simulink model "FTD_test_tau_w"  (R2023a)
settings: Solver=VariableStepAuto  StartTime=0.0  StopTime=150  FixedStep=0.002s  RelTol=1e-3
libraries: simulink x2
settings Model: Creator=邓宇飞  LastModifiedBy=邓宇飞

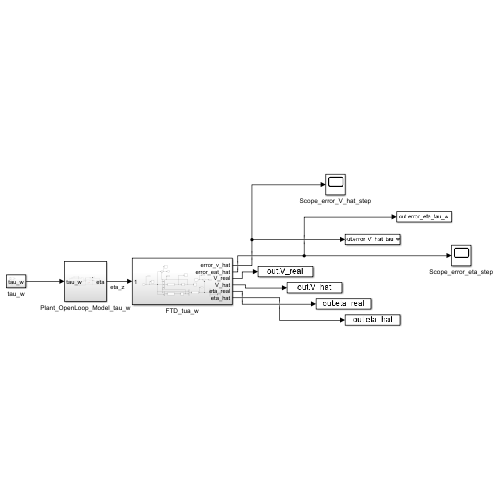
[thumbnail: Simulink's stored preview of the top-level diagram]
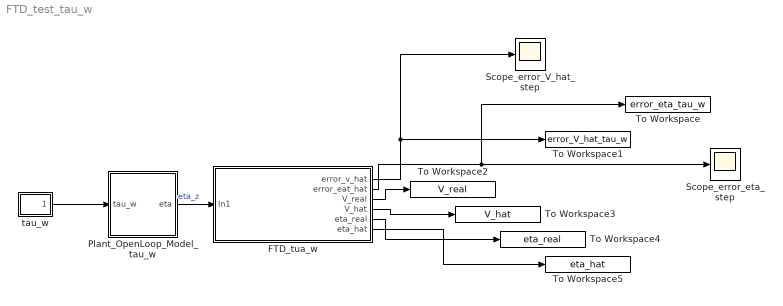
== system FTD_test_tau_w ==
  FTD_tua_w : Subsystem
  Plant_OpenLoop_Model_tau_w : Subsystem
  Scope_error_V_hat_step : Scope
  Scope_error_eta_step : Scope
  To Workspace : ToWorkspace  VariableName=error_eta_tau_w  SaveFormat=Timeseries  SampleTime=-1
  To Workspace1 : ToWorkspace  VariableName=error_V_hat_tau_w  SaveFormat=Timeseries  SampleTime=-1
  To Workspace2 : ToWorkspace  VariableName=V_real  SaveFormat=Timeseries  SampleTime=-1
  To Workspace3 : ToWorkspace  VariableName=V_hat  SaveFormat=Timeseries  SampleTime=-1
  To Workspace4 : ToWorkspace  VariableName=eta_real  SaveFormat=Timeseries  SampleTime=-1
  To Workspace5 : ToWorkspace  VariableName=eta_hat  SaveFormat=Timeseries  SampleTime=-1
  tau_w : Subsystem
  wires:
  FTD_tua_w/2(error_eat_hat) -> To Workspace/1, Scope_error_eta_step/1
  Plant_OpenLoop_Model_tau_w/1(eta) -> FTD_tua_w/1(In1)  "eta_z"
  FTD_tua_w/1(error_v_hat) -> To Workspace1/1, Scope_error_V_hat_step/1
  tau_w/1(tau_w) -> Plant_OpenLoop_Model_tau_w/1(tau_w)
  FTD_tua_w/3(V_real) -> To Workspace2/1
  FTD_tua_w/4(V_hat) -> To Workspace3/1
  FTD_tua_w/5(eta_real) -> To Workspace4/1
  FTD_tua_w/6(eta_hat) -> To Workspace5/1

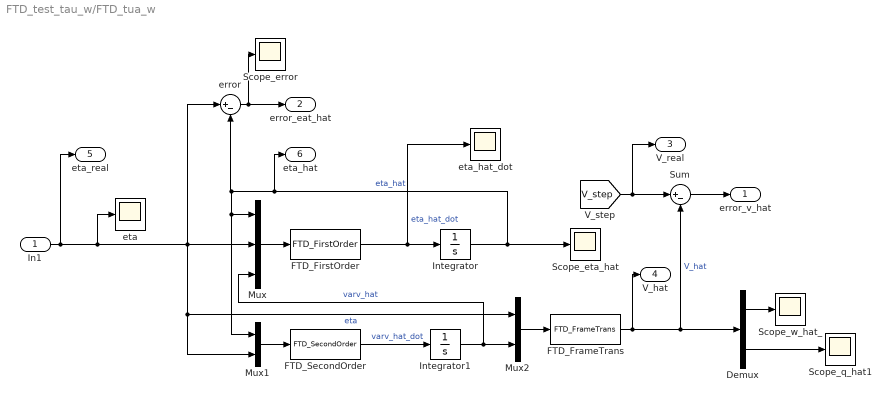
== system FTD_test_tau_w/FTD_tua_w ==
  In1 : Inport
  Demux : Demux  Outputs=2
  FTD_FirstOrder : MATLABFcn  MATLABFcn=FTD_FirstOrder  OutputDimensions=2  OutputSignalType=real
  FTD_FrameTrans : MATLABFcn  MATLABFcn=FTD_FrameTrans  OutputDimensions=2  OutputSignalType=real
  FTD_SecondOrder : MATLABFcn  MATLABFcn=FTD_SecondOrder  OutputDimensions=2  OutputSignalType=real
  Integrator : Integrator
  Integrator1 : Integrator
  Mux : Mux  Inputs=3
  Mux1 : Mux  Inputs=2
  Mux2 : Mux  Inputs=2
  Scope_error : Scope
  Scope_eta_hat : Scope
  Scope_q_hat1 : Scope
  Scope_w_hat_ : Scope
  Sum : Sum  Inputs=|+-
  error : Sum  Inputs=|+-
  eta : Scope
  eta_hat_dot : Scope
  error_v_hat : Outport
  error_eat_hat : Outport  Port=2
  V_real : Outport  Port=3
  V_hat : Outport  Port=4
  eta_real : Outport  Port=5
  eta_hat : Outport  Port=6
  wires:
  In1/1 -> eta_real/1, eta/1, error/1, Mux2/1, Mux1/2, Mux/2  "eta"
  Mux/1 -> FTD_FirstOrder/1
  Integrator/1 -> Scope_eta_hat/1, eta_hat/1, error/2, Mux1/1, Mux/1  "eta_hat"
  FTD_FrameTrans/1 -> V_hat/1, Demux/1, Sum/2  "V_hat"
  FTD_FirstOrder/1 -> Integrator/1, eta_hat_dot/1  "eta_hat_dot"
  error/1 -> error_eat_hat/1, Scope_error/1
  Demux/1 -> Scope_w_hat_/1
  FTD_SecondOrder/1 -> Integrator1/1  "varv_hat_dot"
  Integrator1/1 -> Mux/3, Mux2/2  "varv_hat"
  Mux1/1 -> FTD_SecondOrder/1
  Mux2/1 -> FTD_FrameTrans/1
  Demux/2 -> Scope_q_hat1/1
  [V_step] -> V_real/1, Sum/1
  Sum/1 -> error_v_hat/1

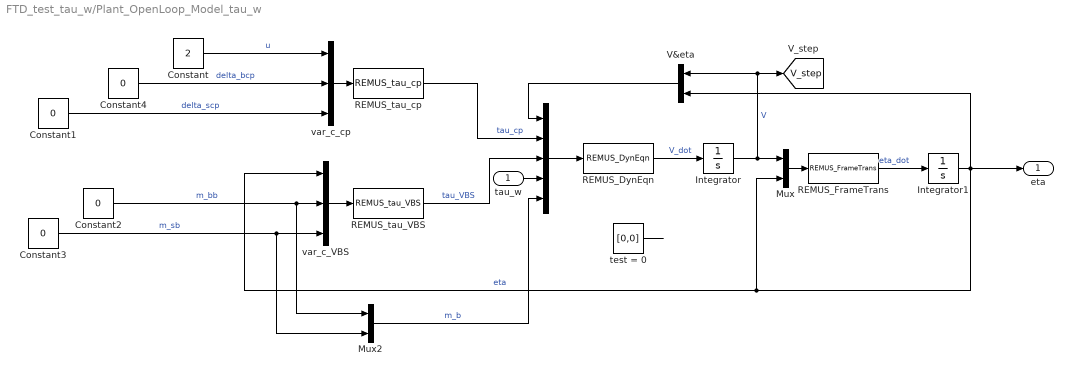
== system FTD_test_tau_w/Plant_OpenLoop_Model_tau_w ==
  tau_w : Inport
  " " : Mux  Inputs=5
  Constant : Constant  Value=2  OutDataTypeStr=Inherit: Inherit via back propagation
  Constant{1..4} (4 alike) : Constant  Value=0
  Integrator : Integrator
  Integrator1 : Integrator
  Mux : Mux  Inputs=2
  Mux2 : Mux  Inputs=2
  REMUS_DynEqn : MATLABFcn  MATLABFcn=REMUS_DynEqn  OutputDimensions=2  OutputSignalType=real
  REMUS_FrameTrans : MATLABFcn  MATLABFcn=REMUS_FrameTrans  OutputDimensions=2  OutputSignalType=real
  REMUS_tau_VBS : MATLABFcn  MATLABFcn=REMUS_tau_VBS  OutputDimensions=2  OutputSignalType=real
  REMUS_tau_cp : MATLABFcn  MATLABFcn=REMUS_tau_cp  OutputDimensions=2  OutputSignalType=real
  V&eta : Mux  Inputs=2
  test = 0 : Constant  Value=[0,0]
  var_c_VBS : Mux  Inputs=3
  var_c_cp : Mux  Inputs=3
  eta : Outport
  tag scope: V_step=global
  wires:
  Constant/1 -> var_c_cp/1  "u"
  REMUS_DynEqn/1 -> Integrator/1  "V_dot"
  REMUS_tau_cp/1 -> " "/2  "tau_cp"
  Integrator1/1 -> eta/1, Mux/2, var_c_VBS/1, V&eta/2  "eta"
  Constant1/1 -> var_c_cp/3  "delta_scp"
  test = 0/1 -> ?
  Constant3/1 -> Mux2/2, var_c_VBS/3  "m_sb"
  Mux/1 -> REMUS_FrameTrans/1
  " "/1 -> REMUS_DynEqn/1
  Integrator/1 -> Mux/1, V&eta/1, [V_step]  "V"
  Constant2/1 -> Mux2/1, var_c_VBS/2  "m_bb"
  Constant4/1 -> var_c_cp/2  "delta_bcp"
  var_c_cp/1 -> REMUS_tau_cp/1
  V&eta/1 -> " "/1
  REMUS_tau_VBS/1 -> " "/3  "tau_VBS"
  tau_w/1 -> " "/4
  REMUS_FrameTrans/1 -> Integrator1/1  "eta_dot"
  var_c_VBS/1 -> REMUS_tau_VBS/1
  Mux2/1 -> " "/5  "m_b"

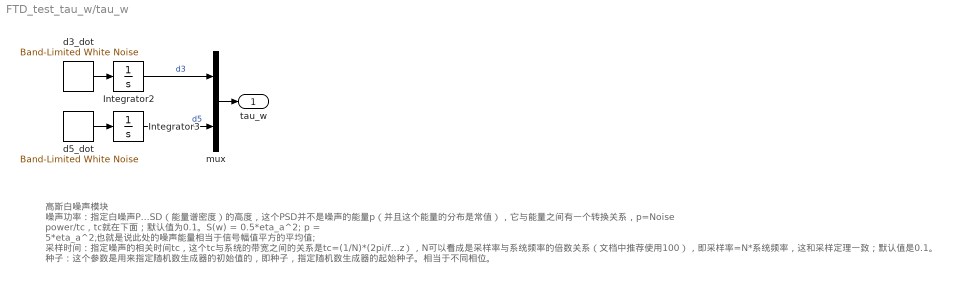
== system FTD_test_tau_w/tau_w ==
  note: 高斯白噪声模块
      | 噪声功率：指定白噪声PSD（能量谱密度）的高度，这个PSD并不是噪声的能量p（并且这个能量的分布是常值），它与能量之间有一个转换关系，p=Noise power/tc，tc就在下面；默认值为0.1。S(w) = 0.5*eta_a^2;
      | p = 5*eta_a^2;也就是说此处的噪声能量相当于信号幅值平方的平均值;
      | 采样时间：指定噪声的相关时间tc，这个tc与系统的带宽之间的关系是tc=(1/N)*(2pi/fmax)，其中fmax是系统的带宽（实际上是角频率，fmax=2*pi*f，这个f才是我们常使用的频率Hz），N可以看成是采样率与系统频率的倍数关系（文档中推荐使用100），即采样率=N*系统频率，这和采样定理一致；默认值是0.1。
      | 种子：这个参数是用来指定随机数生成器的初始值的，即种子，指定随机数生成器的起始种子。相当于不同相位。
  Integrator2 : Integrator
  Integrator3 : Integrator
  d3_dot : simulink/Sources/Band-Limited White Noise  Cov=[0.5]  Ts=0.1  seed=[2]
  d5_dot : simulink/Sources/Band-Limited White Noise  Cov=[0.1]  Ts=0.1  seed=[3]
  mux : Mux  Inputs=2
  tau_w : Outport
  wires:
  Integrator3/1 -> mux/2  "d5"
  d5_dot/1 -> Integrator3/1
  d3_dot/1 -> Integrator2/1
  mux/1 -> tau_w/1
  Integrator2/1 -> mux/1  "d3"
